simulink model "sampleModel1981"  (R2023a)
settings: Solver=VariableStepAuto  StartTime=0.0  StopTime=10.0  RelTol=1e-3
libraries: hdlsllib x4, simulink x3
settings Model: Creator=user1  LastModifiedBy=user1

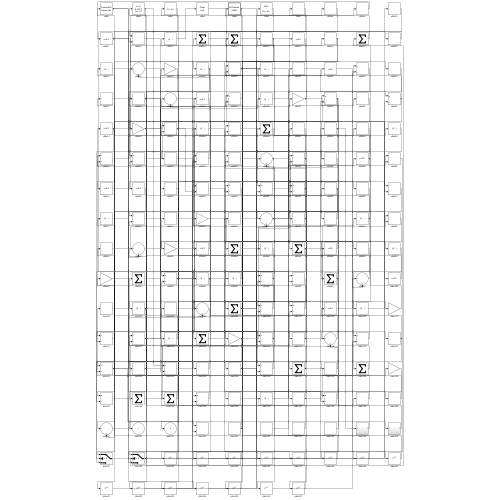
[thumbnail: Simulink's stored preview of the top-level diagram]
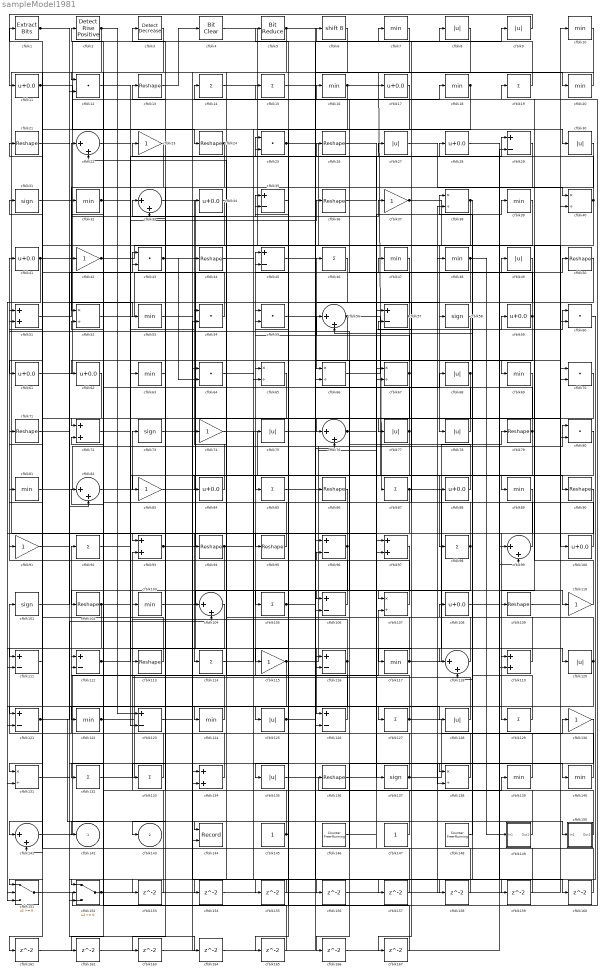
== system sampleModel1981 ==
  cfblk1 : simulink/Logic and Bit Operations/Extract Bits  bitsToExtract=Upper half  numBits=8  bitIdxRange=[0 7]  outScalingMode=Preserve fixed-point scaling
      settings: LibrarySourceBlock=|
      | hdlsllib/Logic and Bit
      | Operations/Extract Bits
  cfblk{7,10,16,18,20,32,39,47..48,53,63,69,81,89,103,117,122,124,139..140} (20 alike) : MinMax
  cfblk{11,17,28,34,41,59,61..62,84,88,100,108} (12 alike) : Bias  Bias=0.0  SaturateOnIntegerOverflow=off
  cfblk{31,58,73,101,137} (5 alike) : Signum
  cfblk{13,21,24,26,36,44,50,71,79,86,90,94..95,102,109,113,136} (17 alike) : Reshape
  cfblk{22,33,56,76,82,99,104,118,141} (9 alike) : Sum  Inputs=|++
  cfblk{14..15,19,46,85,87,92,98,105,114,127,129,132..133} (14 alike) : Sum  Inputs=+
  cfblk{29,35,45,57,96,106,111..112,116,121,123,126} (12 alike) : Sum  Inputs=+-
  cfblk{38,40,52,65..67,107,131,138} (9 alike) : Product  Inputs=*/  RndMeth=Zero  SaturateOnIntegerOverflow=on
  cfblk{23,37,42,74,83,91,110,115,130} (9 alike) : Gain
  cfblk{51,72,93,97,119,134} (6 alike) : Sum
  cfblk{12,25,43,54..55,60,64,70,80} (9 alike) : DotProduct  OutDataTypeStr=Inherit: Inherit via internal rule
  cfblk{8..9,27,30,49,68,75,77..78,120,125,128,135} (13 alike) : Abs  SaturateOnIntegerOverflow=off
  cfblk144 : Record  FileSettingsInternal="{\"entries\":[{\"content\":{\"excelSettings\":{\"content\":{},\"type\":\"Streamout.ExcelSettings\"}},\"type\":\"Streamout.FileSettingStorage\",\"uuid\":\"\"}],\"packageUris\":[\"http:\\/\\/schema.mathworks.com\\/mf0\\/streamout_blocks\\/R2020a\"],\"version\":\"1.0\"}"  Layout=[1 1]  SignalsInternal="{\"entries\":[{\"content\":{\"signals\":[{\"content\":{\"blockPath\":[],\"dimensions\":[1],\"domain\":\"\",\"lineColor\":\"#a2142f\",\"plots\":[1],\"port\":1,\"signalID\":5674,\"signalName\":\"XY Graph:1\"},\"type\":\"RecordBlkView.Signal\",\"uuid\":\"\"},{\"content\":{\"blockPath\":[],\"dimensions\":[1],\"domain\":\"\",\"lineColor\":\"#139fff\",\"plots\":[1],\"port\":2,\"signalID\":5677,\"signalName\":\"XY Graph:2\"},\"type\":\"RecordBlkView.Signal\",\"uuid\":\"\"}]},\"type\":\"RecordBlkView.InputSignals\",\"uuid\":\"\"}],\"packageUris\":[\"http:\\/\\/schema.mathworks.com\\/mf0\\/streamout_blocks\\/R2020a\"],\"version\":\"1.0\"}"  VisualizationBindings="{\"xyplotplugin\":{\"info\":[{\"series\":[{\"bindingParametersList\":[{\"parameter\":\"X-Axis\",\"signalID\":5674,\"signalName\":\"XY Graph:1\"},{\"parameter\":\"Y-Axis\",\"signalID\":5677,\"signalName\":\"XY Graph:2\"}],\"seriesID\":16852}],\"subplotID\":1}]}}"  CompatibilityTag=XY  st=-1
  cfblk145 : Constant  SampleTime=-1
  cfblk146 : hdlsllib/Sources/Counter Free-Running  NumBits=16  tsamp=-1
  cfblk147 : Constant  SampleTime=-1
  cfblk148 : hdlsllib/Sources/Counter Free-Running  NumBits=16  tsamp=-1
  cfblk149 : Subsystem
      settings: LibrarySourceBlock=|
      | hdlsllib/Ports &
      | Subsystems/Subsystem
  cfblk150 : Subsystem
      settings: LibrarySourceBlock=|
      | hdlsllib/Ports &
      | Subsystems/Subsystem
  cfblk151 : Switch  SaturateOnIntegerOverflow=off  InputSameDT=off
  cfblk152 : Switch  SaturateOnIntegerOverflow=off  InputSameDT=off
  cfblk{153..167} (15 alike) : Delay  SampleTime=1
  cfblk2 : hdlsllib/Logic and Bit Operations/Detect Rise Positive  vinit=0  OutDataTypeStr=boolean
  cfblk3 : simulink/Logic and Bit Operations/Detect Decrease  vinit=0.0  OutDataTypeStr=boolean
      settings: LibrarySourceBlock=|
      | hdlsllib/Logic and Bit
      | Operations/Detect
      | Decrease
  cfblk4 : simulink/Logic and Bit Operations/Bit Clear  iBit=0
      settings: LibrarySourceBlock=|
      | hdlsllib/Logic and Bit
      | Operations/Bit Clear
  cfblk5 : hdlsllib/Logic and Bit Operations/Bit Reduce  mode=AND
  cfblk6 : ArithShift  BitShiftNumber=8
  cfblk142 : Outport  VectorParamsAs1DForOutWhenUnconnected=off
  cfblk143 : Outport  Port=2  VectorParamsAs1DForOutWhenUnconnected=off
  wires:
  cfblk13/1 -> cfblk4/1
  cfblk133/1 -> cfblk92/1
  cfblk61/1 -> cfblk18/1
  cfblk121/1 -> cfblk150/1(In1), cfblk51/2, cfblk104/2
  cfblk134/1 -> cfblk101/1
  cfblk2/1 -> cfblk114/1, cfblk123/1
  cfblk106/1 -> cfblk45/1
  cfblk42/1 -> cfblk78/1, cfblk36/1
  cfblk124/1 -> cfblk112/1
  cfblk111/1 -> cfblk41/1
  cfblk33/1 -> cfblk76/1
  cfblk16/1 -> cfblk87/1, cfblk105/1, cfblk165/1
  cfblk10/1 -> cfblk111/1
  cfblk40/1 -> cfblk23/1, cfblk109/1
  cfblk19/1 -> cfblk6/1
  cfblk88/1 -> cfblk51/1
  cfblk29/1 -> cfblk102/1
  cfblk90/1 -> cfblk129/1
  cfblk141/1 -> cfblk65/1
  cfblk81/1 -> cfblk80/1
  cfblk14/1 -> cfblk137/1
  cfblk104/1 -> cfblk141/1
  cfblk31/1 -> cfblk9/1
  cfblk65/1 -> cfblk142/1
  cfblk83/1 -> cfblk126/1
  cfblk54/1 -> cfblk31/1
  cfblk77/1 -> cfblk25/1, cfblk95/1
  cfblk135/1 -> cfblk139/1
  cfblk115/1 -> cfblk48/1, cfblk152/3
  cfblk145/1 -> cfblk3/1, cfblk5/1
  cfblk146/1 -> cfblk97/1
  cfblk4/1 -> cfblk76/2
  cfblk20/1 -> cfblk17/1
  cfblk41/1 -> cfblk35/1, cfblk121/2
  cfblk127/1 -> cfblk130/1, cfblk96/2
  cfblk45/1 -> cfblk66/1
  cfblk5/1 -> cfblk122/1, cfblk80/2
  cfblk51/1 -> cfblk22/1
  cfblk49/1 -> cfblk115/1
  cfblk94/1 -> cfblk138/2, cfblk163/1
  cfblk11/1 -> cfblk24/1, cfblk82/2
  cfblk113/1 -> cfblk91/1
  cfblk107/1 -> cfblk21/1
  cfblk82/1 -> cfblk73/1
  cfblk56/1 -> cfblk99/2, cfblk133/1
  cfblk93/1 -> cfblk50/1, cfblk156/1
  cfblk118/1 -> cfblk35/2
  cfblk69/1 -> cfblk77/1
  cfblk46/1 -> cfblk132/1
  cfblk78/1 -> cfblk2/1
  cfblk117/1 -> cfblk79/1, cfblk22/2
  cfblk3/1 -> cfblk12/1
  cfblk34/1 -> cfblk141/2
  cfblk24/1 -> cfblk143/1, cfblk72/1
  cfblk73/1 -> cfblk34/1
  cfblk23/1 -> cfblk52/1
  cfblk75/1 -> cfblk46/1
  cfblk43/1 -> cfblk136/1, cfblk64/2
  cfblk86/1 -> cfblk111/2
  cfblk1/1 -> cfblk128/1, cfblk138/1
  cfblk91/1 -> cfblk124/1
  cfblk37/1 -> cfblk7/1, cfblk100/1
  cfblk89/1 -> cfblk135/1
  cfblk55/1 -> cfblk58/1
  cfblk68/1 -> cfblk127/1, cfblk116/2
  cfblk60/1 -> cfblk152/1
  cfblk38/1 -> cfblk42/1, cfblk158/1, cfblk161/1
  cfblk87/1 -> cfblk119/1, cfblk126/2
  cfblk151/1 -> cfblk19/1
  cfblk52/1 -> cfblk47/1
  cfblk84/1 -> cfblk44/1
  cfblk96/1 -> cfblk93/1, cfblk125/1
  cfblk57/1 -> cfblk106/1, cfblk26/1
  cfblk47/1 -> cfblk61/1
  cfblk103/1 -> cfblk110/1
  cfblk66/1 -> cfblk59/1
  cfblk100/1 -> cfblk13/1
  cfblk149/1(Out1) -> cfblk43/1
  cfblk12/1 -> cfblk97/2
  cfblk123/1 -> cfblk64/1
  cfblk137/1 -> cfblk119/2, cfblk55/2
  cfblk76/1 -> cfblk39/1, cfblk49/1
  cfblk138/1 -> cfblk71/1
  cfblk126/1 -> cfblk74/1
  cfblk110/1 -> cfblk14/1
  cfblk147/1 -> cfblk93/2
  cfblk67/1 -> cfblk62/1, cfblk55/1, cfblk151/1, cfblk155/1
  cfblk105/1 -> cfblk68/1, cfblk8/1
  cfblk116/1 -> cfblk103/1, cfblk151/3
  cfblk79/1 -> cfblk27/1, cfblk123/2
  cfblk44/1 -> cfblk90/1
  cfblk92/1 -> cfblk118/1
  cfblk101/1 -> cfblk43/2
  cfblk128/1 -> cfblk113/1
  cfblk35/1 -> cfblk15/1
  cfblk22/1 -> cfblk63/1
  cfblk72/1 -> cfblk37/1
  cfblk119/1 -> cfblk33/1
  cfblk59/1 -> cfblk16/1, cfblk83/1
  cfblk9/1 -> cfblk11/1
  cfblk95/1 -> cfblk33/2
  cfblk80/1 -> cfblk98/1
  cfblk102/1 -> cfblk28/1, cfblk151/2
  cfblk136/1 -> cfblk60/1
  cfblk6/1 -> cfblk12/2
  cfblk58/1 -> cfblk107/1
  cfblk148/1 -> cfblk108/1
  cfblk74/1 -> cfblk89/1
  cfblk25/1 -> cfblk70/1, cfblk70/2, cfblk30/1
  cfblk27/1 -> cfblk40/1
  cfblk17/1 -> cfblk131/1
  cfblk50/1 -> cfblk85/1
  cfblk112/1 -> cfblk54/1, cfblk120/1
  cfblk139/1 -> cfblk81/1
  cfblk122/1 -> cfblk107/2, cfblk52/2
  cfblk140/1 -> cfblk82/1
  cfblk109/1 -> cfblk10/1
  cfblk131/1 -> cfblk144/1
  cfblk99/1 -> cfblk57/2
  cfblk21/1 -> cfblk53/1
  cfblk120/1 -> cfblk38/1, cfblk131/2
  cfblk98/1 -> cfblk32/1, cfblk162/1
  cfblk129/1 -> cfblk56/2
  cfblk26/1 -> cfblk69/1
  cfblk18/1 -> cfblk65/2, cfblk134/2
  cfblk114/1 -> cfblk75/1
  cfblk15/1 -> cfblk20/1
  cfblk152/1 -> cfblk96/1, cfblk38/2
  cfblk150/1(Out1) -> cfblk118/2
  cfblk7/1 -> cfblk84/1
  cfblk85/1 -> cfblk67/1
  cfblk53/1 -> cfblk88/1
  cfblk132/1 -> cfblk86/1
  cfblk48/1 -> cfblk117/1, cfblk149/1(In1)
  cfblk8/1 -> cfblk144/2
  cfblk62/1 -> cfblk121/1
  cfblk125/1 -> cfblk140/1, cfblk157/1
  cfblk36/1 -> cfblk29/1
  cfblk108/1 -> cfblk29/2
  cfblk30/1 -> cfblk67/2
  cfblk39/1 -> cfblk104/1
  cfblk32/1 -> cfblk116/1, cfblk94/1
  cfblk63/1 -> cfblk153/1
  cfblk153/1 -> cfblk112/2
  cfblk97/1 -> cfblk154/1
  cfblk154/1 -> cfblk40/2
  cfblk155/1 -> cfblk152/2
  cfblk156/1 -> cfblk60/2
  cfblk157/1 -> cfblk1/1
  cfblk158/1 -> cfblk45/2
  cfblk64/1 -> cfblk159/1
  cfblk159/1 -> cfblk56/1
  cfblk28/1 -> cfblk160/1
  cfblk160/1 -> cfblk57/1
  cfblk161/1 -> cfblk134/1
  cfblk162/1 -> cfblk54/2
  cfblk163/1 -> cfblk66/2
  cfblk71/1 -> cfblk164/1
  cfblk164/1 -> cfblk106/2
  cfblk165/1 -> cfblk72/2
  cfblk130/1 -> cfblk166/1
  cfblk166/1 -> cfblk99/1
  cfblk70/1 -> cfblk167/1
  cfblk167/1 -> cfblk25/2

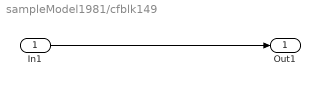
== system sampleModel1981/cfblk149 ==
  In1 : Inport
  Out1 : Outport
  wires:
  In1/1 -> Out1/1

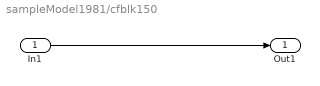
== system sampleModel1981/cfblk150 ==
  In1 : Inport
  Out1 : Outport
  wires:
  In1/1 -> Out1/1
